simulink model "PI_graph"  (R2024b)
settings: Solver=VariableStepAuto  StartTime=0.0  StopTime=10.0  RelTol=1e-3
values from neighbouring files (symbols this model uses):
  K = PHT/(H_aux*PHT + diag(matR(ind_z)))    [EKF_IMU.m]    (also in EKF_NAV.m; EKF_WFL.m; PID_MV.m = PARAM.K; SFC.m = PARAM.K)
  Ti = PARAM.Ti    [PID_MV.m]
settings Model: Creator=diego-ubuntu  LastModifiedBy=diego-ubuntu

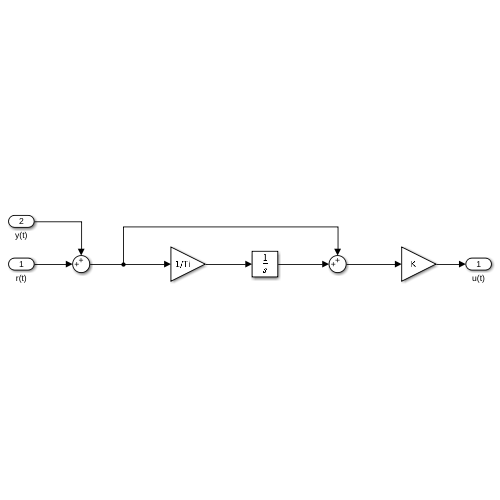
[thumbnail: Simulink's stored preview of the top-level diagram]
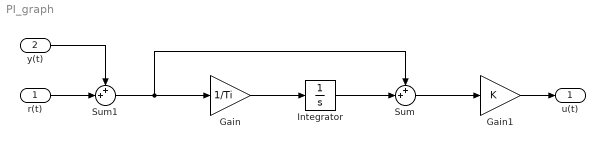
== system PI_graph ==
  r(t) : Inport
  y(t) : Inport  Port=2
  Gain : Gain  Gain=1/Ti
  Gain1 : Gain  Gain=K
  Integrator : Integrator
  Sum : Sum  Inputs=++|
  Sum1 : Sum  Inputs=++|
  u(t) : Outport
  wires:
  Sum/1 -> Gain1/1
  Gain/1 -> Integrator/1
  Sum1/1 -> Sum/1, Gain/1
  Gain1/1 -> u(t)/1
  Integrator/1 -> Sum/2
  r(t)/1 -> Sum1/2
  y(t)/1 -> Sum1/1
